simulink model "helicopter_p"  (R2022a)
settings: Solver=VariableStepAuto  StartTime=0.0  StopTime=3  RelTol=1e-3
model workspace (MATLAB code in the model file):
  | I_yy = 20;
  | K = 100;
  | b = 5;
  | init_vel = 0;
  | inverse_I_yy = 1/I_yy;
  | inverse_K = 1/K;
settings Model: Creator=ba13  LastModifiedBy=ba13

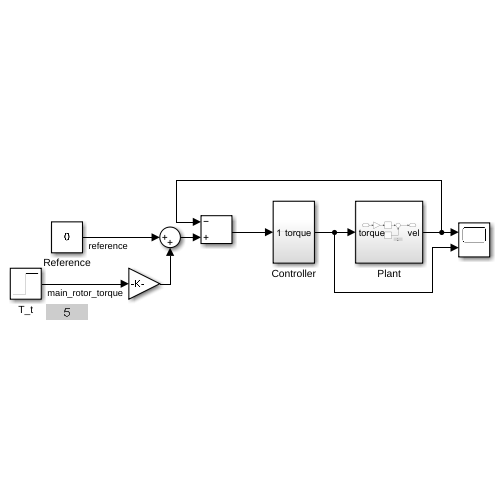
[thumbnail: Simulink's stored preview of the top-level diagram]
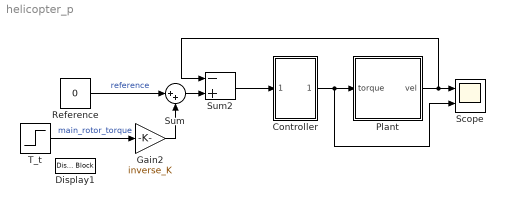
== system helicopter_p ==
  Controller : Subsystem
  Display1 : DisplayBlock  LabelPosition=Hide  Transparency=1
  Gain2 : Gain  Gain=inverse_K
  Plant : Subsystem
  Reference : Constant  Value=0
  Scope : Scope  NumInputPorts=2
  Sum : Sum  Inputs=|++
  Sum2 : Sum  Inputs=-+
  T_t : Step  After=b  SampleTime=0
  wires:
  Reference/1 -> Sum/1  "reference"
  Sum/1 -> Sum2/2
  T_t/1 -> Gain2/1  "main_rotor_torque"
  Gain2/1 -> Sum/2
  Plant/1(vel) -> Scope/1, Sum2/1
  Controller/1(torque) -> Scope/2, Plant/1(torque)
  Sum2/1 -> Controller/1(In1)

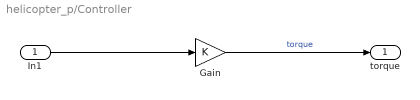
== system helicopter_p/Controller ==
  In1 : Inport
  Gain : Gain  Gain=K
  torque : Outport
  wires:
  Gain/1 -> torque/1  "torque"
  In1/1 -> Gain/1

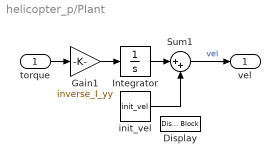
== system helicopter_p/Plant ==
  torque : Inport
  Display : DisplayBlock  LabelPosition=Hide  Transparency=1
  Gain1 : Gain  Gain=inverse_I_yy
  Integrator : Integrator
  Sum1 : Sum  Inputs=|++
  init_vel : Constant  Value=init_vel
  vel : Outport
  wires:
  Integrator/1 -> Sum1/1
  Gain1/1 -> Integrator/1
  init_vel/1 -> Sum1/2
  torque/1 -> Gain1/1
  Sum1/1 -> vel/1  "vel"
